simulink model "Subsystems"  (R2021b)
settings: Solver=ode4  StartTime=0.0  StopTime=10.0  FixedStep=10^-5  RelTol=1e-3
undefined symbols (not defined in the file): sigbuilder_block
settings Model: Creator=amr_y  LastModifiedBy=amr_y

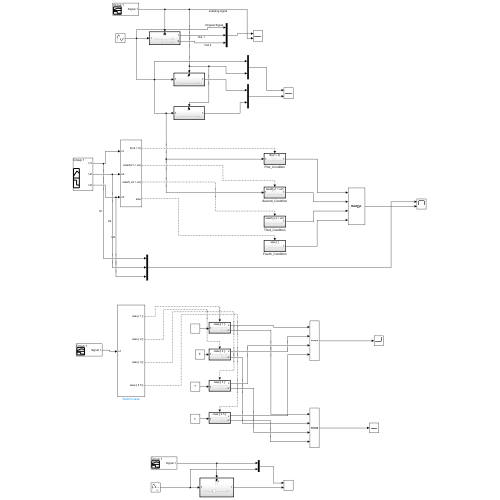
[thumbnail: Simulink's stored preview of the top-level diagram]
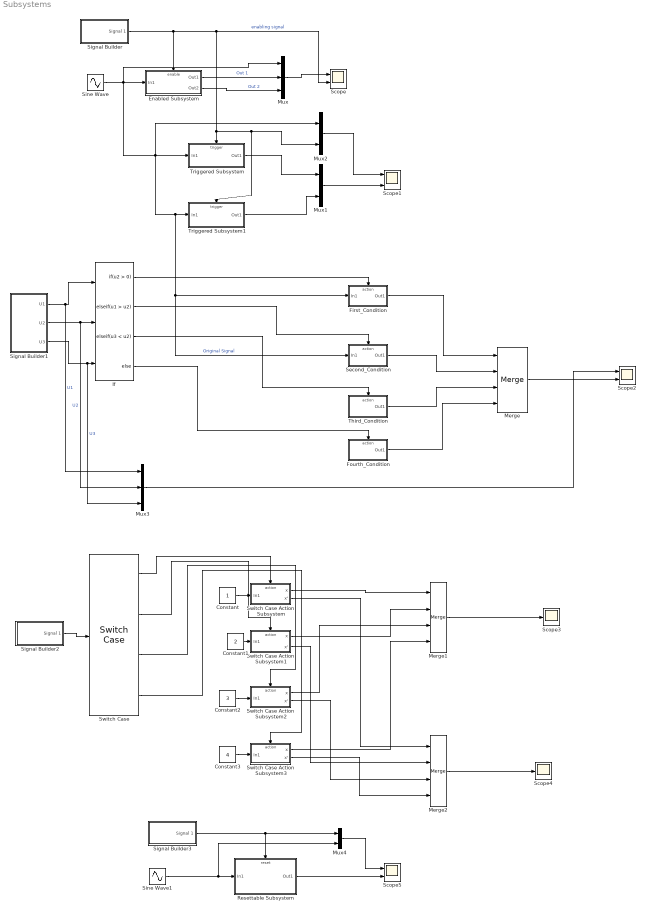
== system Subsystems ==
  Constant : Constant
  Constant1 : Constant  Value=2
  Constant2 : Constant  Value=3
  Constant3 : Constant  Value=4
  Enabled Subsystem : Subsystem  TreatAsAtomicUnit=on
  First_Condition : Subsystem  TreatAsAtomicUnit=on
  Fourth_Condition : Subsystem  TreatAsAtomicUnit=on
  If : If  NumInputs=3  IfExpression=u2 > 0  ElseIfExpressions=u1 > u2, u3 < u2
  Merge : Merge  Inputs=4  InitialOutput=0
  Merge1 : Merge  Inputs=4  InitialOutput=4
  Merge2 : Merge  Inputs=4  InitialOutput=-1
  Mux : Mux  Inputs=3
  Mux1 : Mux  Inputs=2
  Mux2 : Mux  Inputs=2
  Mux3 : Mux  Inputs=3
  Mux4 : Mux  Inputs=2
  Resettable Subsystem : Subsystem  TreatAsAtomicUnit=on
  Scope{,1..2,5} (4 alike) : Scope  NumInputPorts=2
  Scope3 : Scope
  Scope4 : Scope
  Second_Condition : Subsystem  TreatAsAtomicUnit=on
  Signal Builder : Subsystem  Tag=STV Subsys  LoadFcn=sigbuilder_block('load');  StartFcn=sigbuilder_block('start');  StopFcn=sigbuilder_block('stop');  ClipboardFcn=sigbuilder_block('clipboard');  mask(Sigbuilder block){tuvar=[0:10]}
      mask help: Simulink:masks:SigbuilderBlock_MD
      mask init:
      | if ~strcmp(get_param(bdroot(gcbh),'SimulationStatus'),'stopped') tuvar = sigbuilder_block('maskInit'); end
      settings: CopyFcn=sigbuilder_block('copy');  DeleteFcn=sigbuilder_block('delete');  ModelCloseFcn=sigbuilder_block('modelClose');  PreSaveFcn=sigbuilder_block('preSave');  PauseFcn=sigbuilder_block('pause');  ContinueFcn=sigbuilder_block('continue');  NameChangeFcn=sigbuilder_block('namechange');  OpenFcn=sigbuilder_block('open',[5.4 30 1141.2 522.6 ]);  CloseFcn=sigbuilder_block('close');
      mask Display: plot(0, 0, 100, 100,[2, 2, 32, 32, 2], [68, 8, 8, 68, 68],[32, 2], [38, 38], [32, 19, 2],[53, 60, 44], [32, 17, 17, 2],[16, 16, 31, 31]);txt = getActiveGroup(gcbh);text(2, 100, txt,'verticalAlignment', 'top');
  Signal Builder1 : Subsystem  Tag=STV Subsys  LoadFcn=sigbuilder_block('load');  StartFcn=sigbuilder_block('start');  StopFcn=sigbuilder_block('stop');  ClipboardFcn=sigbuilder_block('clipboard');  mask(Sigbuilder block){tuvar=[0:10]}
      mask help: Simulink:masks:SigbuilderBlock_MD
      mask init:
      | if ~strcmp(get_param(bdroot(gcbh),'SimulationStatus'),'stopped') tuvar = sigbuilder_block('maskInit'); end
      settings: CopyFcn=sigbuilder_block('copy');  DeleteFcn=sigbuilder_block('delete');  ModelCloseFcn=sigbuilder_block('modelClose');  PreSaveFcn=sigbuilder_block('preSave');  PauseFcn=sigbuilder_block('pause');  ContinueFcn=sigbuilder_block('continue');  NameChangeFcn=sigbuilder_block('namechange');  OpenFcn=sigbuilder_block('open',[0 30 1152 561.6 ]);  CloseFcn=sigbuilder_block('close');
      mask Display: plot(0, 0, 100, 100,[2, 2, 32, 32, 2], [68, 8, 8, 68, 68],[32, 2], [38, 38], [32, 19, 2],[53, 60, 44], [32, 17, 17, 2],[16, 16, 31, 31]);txt = getActiveGroup(gcbh);text(2, 100, txt,'verticalAlignment', 'top');
  Signal Builder2 : Subsystem  Tag=STV Subsys  LoadFcn=sigbuilder_block('load');  StartFcn=sigbuilder_block('start');  StopFcn=sigbuilder_block('stop');  ClipboardFcn=sigbuilder_block('clipboard');  mask(Sigbuilder block){tuvar=[0:10]}
      mask help: Simulink:masks:SigbuilderBlock_MD
      mask init:
      | if ~strcmp(get_param(bdroot(gcbh),'SimulationStatus'),'stopped') tuvar = sigbuilder_block('maskInit'); end
      settings: CopyFcn=sigbuilder_block('copy');  DeleteFcn=sigbuilder_block('delete');  ModelCloseFcn=sigbuilder_block('modelClose');  PreSaveFcn=sigbuilder_block('preSave');  PauseFcn=sigbuilder_block('pause');  ContinueFcn=sigbuilder_block('continue');  NameChangeFcn=sigbuilder_block('namechange');  OpenFcn=sigbuilder_block('open',[5.4 30 1141.2 522.6 ]);  CloseFcn=sigbuilder_block('close');
      mask Display: plot(0, 0, 100, 100,[2, 2, 32, 32, 2], [68, 8, 8, 68, 68],[32, 2], [38, 38], [32, 19, 2],[53, 60, 44], [32, 17, 17, 2],[16, 16, 31, 31]);txt = getActiveGroup(gcbh);text(2, 100, txt,'verticalAlignment', 'top');
  Signal Builder3 : Subsystem  Tag=STV Subsys  LoadFcn=sigbuilder_block('load');  StartFcn=sigbuilder_block('start');  StopFcn=sigbuilder_block('stop');  ClipboardFcn=sigbuilder_block('clipboard');  mask(Sigbuilder block){tuvar=[0:10]}
      mask help: Simulink:masks:SigbuilderBlock_MD
      mask init:
      | if ~strcmp(get_param(bdroot(gcbh),'SimulationStatus'),'stopped') tuvar = sigbuilder_block('maskInit'); end
      settings: CopyFcn=sigbuilder_block('copy');  DeleteFcn=sigbuilder_block('delete');  ModelCloseFcn=sigbuilder_block('modelClose');  PreSaveFcn=sigbuilder_block('preSave');  PauseFcn=sigbuilder_block('pause');  ContinueFcn=sigbuilder_block('continue');  NameChangeFcn=sigbuilder_block('namechange');  OpenFcn=sigbuilder_block('open',[437.6 199.2 550.4 400 ]);  CloseFcn=sigbuilder_block('close');
      mask Display: plot(0, 0, 100, 100,[2, 2, 32, 32, 2], [68, 8, 8, 68, 68],[32, 2], [38, 38], [32, 19, 2],[53, 60, 44], [32, 17, 17, 2],[16, 16, 31, 31]);txt = getActiveGroup(gcbh);text(2, 100, txt,'verticalAlignment', 'top');
  Sine Wave : Sin  SampleTime=0
  Sine Wave1 : Sin  SampleTime=0
  Switch Case : SwitchCase  CaseConditions={1,2,3,[4,5]}  ShowDefaultCase=off
  Switch Case Action Subsystem : Subsystem  TreatAsAtomicUnit=on
  Switch Case Action Subsystem1 : Subsystem  TreatAsAtomicUnit=on
  Switch Case Action Subsystem2 : Subsystem  TreatAsAtomicUnit=on
  Switch Case Action Subsystem3 : Subsystem  TreatAsAtomicUnit=on
  Third_Condition : Subsystem  TreatAsAtomicUnit=on
  Triggered Subsystem : Subsystem  TreatAsAtomicUnit=on
  Triggered Subsystem1 : Subsystem  TreatAsAtomicUnit=on
  wires:
  Sine Wave/1 -> Mux2/1, Second_Condition/1(In1), First_Condition/1(In1), Triggered Subsystem1/1(In1), Triggered Subsystem/1(In1), Mux/1, Enabled Subsystem/1(In1)  "Original Signal"
  Signal Builder/1(Signal 1) -> Scope/2, Triggered Subsystem1/Trigger, Mux2/2, Triggered Subsystem/Trigger, Enabled Subsystem/Enable  "enabling signal"
  Mux/1 -> Scope/1
  Enabled Subsystem/1(Out1) -> Mux/2  "Out 1"
  Enabled Subsystem/2(Out2) -> Mux/3  "Out 2"
  Triggered Subsystem/1(Out1) -> Mux1/1
  Triggered Subsystem1/1(Out1) -> Mux1/2
  Mux1/1 -> Scope1/2
  Mux2/1 -> Scope1/1
  If/2 -> Second_Condition/Action
  If/3 -> Third_Condition/Action
  If/4 -> Fourth_Condition/Action
  Second_Condition/1(Out1) -> Merge/2
  First_Condition/1(Out1) -> Merge/1
  Third_Condition/1(Out1) -> Merge/3
  Fourth_Condition/1(Out1) -> Merge/4
  Merge/1 -> Scope2/2
  Signal Builder1/1(U1) -> Mux3/1, If/1  "U1"
  Signal Builder1/2(U2) -> Mux3/2, If/2  "U2"
  Signal Builder1/3(U3) -> Mux3/3, If/3  "U3"
  If/1 -> First_Condition/Action
  Mux3/1 -> Scope2/1
  Switch Case/1 -> Switch Case Action Subsystem/Action
  Switch Case/2 -> Switch Case Action Subsystem1/Action
  Switch Case/3 -> Switch Case Action Subsystem2/Action
  Switch Case/4 -> Switch Case Action Subsystem3/Action
  Switch Case Action Subsystem/1(x) -> Merge1/1
  Switch Case Action Subsystem1/1(x) -> Merge1/2
  Switch Case Action Subsystem2/1(x) -> Merge1/3
  Switch Case Action Subsystem3/1(x) -> Merge1/4
  Switch Case Action Subsystem/2(x') -> Merge2/1
  Switch Case Action Subsystem1/2(x') -> Merge2/2
  Switch Case Action Subsystem2/2(x') -> Merge2/3
  Switch Case Action Subsystem3/2(x') -> Merge2/4
  Signal Builder2/1(Signal 1) -> Switch Case/1
  Constant/1 -> Switch Case Action Subsystem/1(In1)
  Constant1/1 -> Switch Case Action Subsystem1/1(In1)
  Constant2/1 -> Switch Case Action Subsystem2/1(In1)
  Constant3/1 -> Switch Case Action Subsystem3/1(In1)
  Merge1/1 -> Scope3/1
  Merge2/1 -> Scope4/1
  Sine Wave1/1 -> Mux4/2, Resettable Subsystem/1(In1)
  Signal Builder3/1(Signal 1) -> Resettable Subsystem/Reset, Mux4/1
  Mux4/1 -> Scope5/1
  Resettable Subsystem/1(Out1) -> Scope5/2

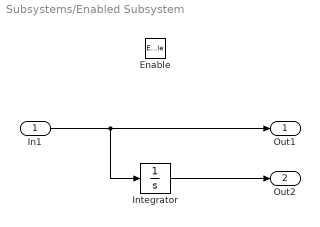
== system Subsystems/Enabled Subsystem ==
  In1 : Inport
  Enable : EnablePort
  Integrator : Integrator
  Out1 : Outport  OutputWhenDisabled=reset  InitialOutput=[0]
  Out2 : Outport  Port=2  OutputWhenDisabled=reset  InitialOutput=[0]
  wires:
  In1/1 -> Integrator/1, Out1/1
  Integrator/1 -> Out2/1

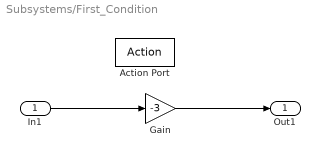
== system Subsystems/First_Condition ==
  In1 : Inport
  Action Port : ActionPort  ActionPortLabel=if(u2 > 0)
  Gain : Gain  Gain=-3
  Out1 : Outport
  wires:
  In1/1 -> Gain/1
  Gain/1 -> Out1/1

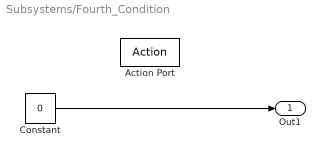
== system Subsystems/Fourth_Condition ==
  Action Port : ActionPort  ActionPortLabel=else
  Constant : Constant  Value=0
  Out1 : Outport
  wires:
  Constant/1 -> Out1/1

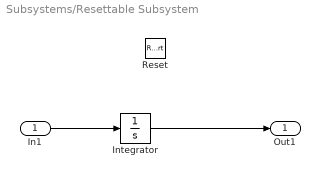
== system Subsystems/Resettable Subsystem ==
  In1 : Inport
  Reset : ResetPort  DisableCoverage=on
  Integrator : Integrator  InitialCondition=3
  Out1 : Outport
  wires:
  In1/1 -> Integrator/1
  Integrator/1 -> Out1/1

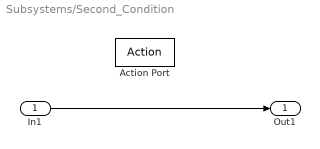
== system Subsystems/Second_Condition ==
  In1 : Inport
  Action Port : ActionPort  ActionPortLabel=elseif(u1 > u2)
  Out1 : Outport
  wires:
  In1/1 -> Out1/1

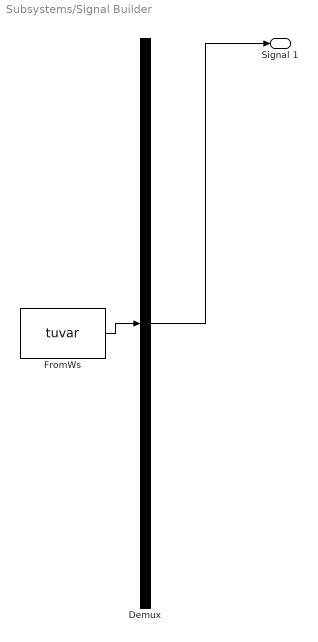
== system Subsystems/Signal Builder ==
  Demux : Demux  Tag=STV Demux  Outputs=1
      settings: DisplayOption=none
  FromWs : FromWorkspace  Tag=STV FromWs  VariableName=tuvar
      SigBuilderData=|
      | common.afterFinalStr = 'Extrapolate'
      | common.sampleTime = 0
      | dataSet.timeRange = [0 10]
      | dataSet.name = 'Group 1'
      | sbobj.Groups.Name = 'Group 1'
      | sbobj.Groups.Signals.Name = 'Signal 1'
      | sbobj.Groups.Signals.XData = [0 2 2 4 4 7 7 9 9 10]
      | sbobj.Groups.Signals.YData = [0 0 1 1 0 0 1 1 0 0]
  Signal 1 : Outport  Tag=STV Outport
  wires:
  Demux/1 -> Signal 1/1
  FromWs/1 -> Demux/1

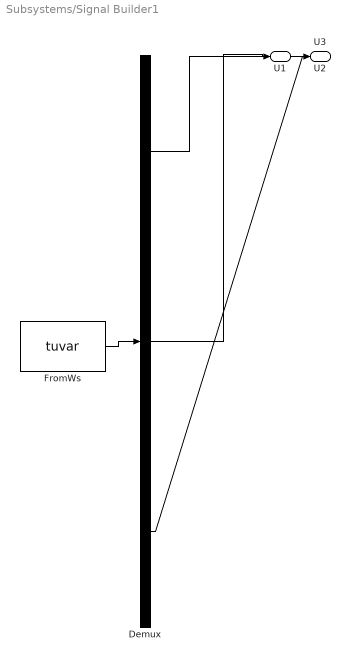
== system Subsystems/Signal Builder1 ==
  Demux : Demux  Tag=STV Demux  Outputs=3
      settings: DisplayOption=none
  FromWs : FromWorkspace  Tag=STV FromWs  VariableName=tuvar
      SigBuilderData=|
      | common.afterFinalStr = 'Extrapolate'
      | common.sampleTime = 0
      | dataSet.timeRange = [0 10]
      | dataSet.name = 'Group 1'
      | sbobj.Groups.Name = 'Group 1'
      | sbobj.Groups.Signals(1).Name = 'U1'
      | sbobj.Groups.Signals(1).XData = [0 3 3 6 6 10]
      | sbobj.Groups.Signals(1).YData = [0 0 1 1 -2 -2]
      | sbobj.Groups.Signals(2).Name = 'U2'
      | sbobj.Groups.Signals(2).XData = [0 3 3 10]
      | sbobj.Groups.Signals(2).YData = [1 1 -1 -1]
      | sbobj.Groups.Signals(3).Name = 'U3'
      | sbobj.Groups.Signals(3).XData = [0 3 3 6 6 8 8 10]
      | sbobj.Groups.Signals(3).YData = [2 2 0 0 -2 -2 0 0]
  U1 : Outport  Tag=STV Outport
  U2 : Outport  Tag=STV Outport  Port=2
  U3 : Outport  Tag=STV Outport  Port=3
  wires:
  Demux/1 -> U1/1
  FromWs/1 -> Demux/1
  Demux/2 -> U2/1
  Demux/3 -> U3/1

== system Subsystems/Signal Builder2 ==
  Demux : Demux  Tag=STV Demux  Outputs=1
      settings: DisplayOption=none
  FromWs : FromWorkspace  Tag=STV FromWs  VariableName=tuvar
      SigBuilderData=|
      | common.afterFinalStr = 'Extrapolate'
      | common.sampleTime = 0
      | dataSet.timeRange = [0 10]
      | dataSet.name = 'Group 1'
      | sbobj.Groups.Name = 'Group 1'
      | sbobj.Groups.Signals.Name = 'Signal 1'
      | sbobj.Groups.Signals.XData = [0 2 2 4 4 6 6 8 8 10]
      | sbobj.Groups.Signals.YData = [1 1 2 2 3 3 4 4 5 5]
  Signal 1 : Outport  Tag=STV Outport
  wires:
  Demux/1 -> Signal 1/1
  FromWs/1 -> Demux/1

== system Subsystems/Signal Builder3 ==
  Demux : Demux  Tag=STV Demux  Outputs=1
      settings: DisplayOption=none
  FromWs : FromWorkspace  Tag=STV FromWs  VariableName=tuvar
      SigBuilderData=|
      | common.afterFinalStr = 'Extrapolate'
      | common.sampleTime = 0
      | dataSet.timeRange = [0 10]
      | dataSet.name = 'Group 1'
      | sbobj.Groups.Name = 'Group 1'
      | sbobj.Groups.Signals.Name = 'Signal 1'
      | sbobj.Groups.Signals.XData = [0 4 4 6 6 10]
      | sbobj.Groups.Signals.YData = [0 0 1 1 0 0]
  Signal 1 : Outport  Tag=STV Outport
  wires:
  Demux/1 -> Signal 1/1
  FromWs/1 -> Demux/1

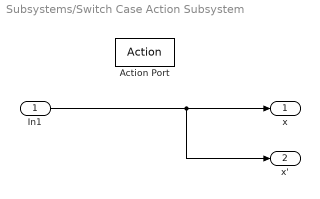
== system Subsystems/Switch Case Action Subsystem ==
  In1 : Inport
  Action Port : ActionPort  ActionPortLabel=case [ 1 ]:
  x : Outport
  x' : Outport  Port=2
  wires:
  In1/1 -> x'/1, x/1

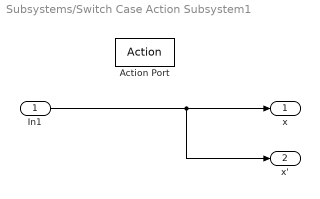
== system Subsystems/Switch Case Action Subsystem1 ==
  In1 : Inport
  Action Port : ActionPort  ActionPortLabel=case [ 2 ]:
  x : Outport
  x' : Outport  Port=2
  wires:
  In1/1 -> x'/1, x/1

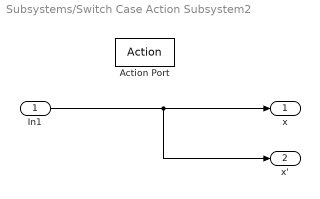
== system Subsystems/Switch Case Action Subsystem2 ==
  In1 : Inport
  Action Port : ActionPort  ActionPortLabel=case [ 3 ]:
  x : Outport
  x' : Outport  Port=2
  wires:
  In1/1 -> x'/1, x/1

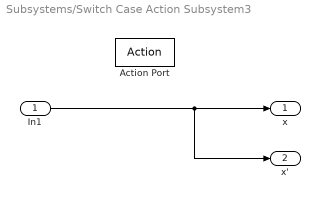
== system Subsystems/Switch Case Action Subsystem3 ==
  In1 : Inport
  Action Port : ActionPort  ActionPortLabel=case [ 4 5 ]:
  x : Outport
  x' : Outport  Port=2
  wires:
  In1/1 -> x'/1, x/1

== system Subsystems/Third_Condition ==
  Action Port : ActionPort  ActionPortLabel=elseif( u3 < u2)
  Constant : Constant  Value=4
  Out1 : Outport
  wires:
  Constant/1 -> Out1/1

== system Subsystems/Triggered Subsystem ==
  In1 : Inport
  Trigger : TriggerPort  VariantControl=(inherit)
  Out1 : Outport
  wires:
  In1/1 -> Out1/1

== system Subsystems/Triggered Subsystem1 ==
  In1 : Inport
  Trigger : TriggerPort  TriggerType=falling  VariantControl=(inherit)
  Out1 : Outport
  wires:
  In1/1 -> Out1/1
